simulink model "yoyo3"  (R2013b)
settings: Solver=ode45  StartTime=0.0  StopTime=10.0  RelTol=1e-3
values from neighbouring files (symbols this model uses):
  H = 1    [yoyo_model.m]    (also in yoyo_model_simulate.m = -100; yoyo_model_testing_lqi.m)
  K = 1    [yoyo_model.m]    (also in yoyo_model_simulate.m = 0.001; yoyo_model_testing_lqi.m)
  phi = fPHI(T,2*T,PARAMS)    [yoyo_model.m]    (also in yoyo_model_simulate.m; yoyo_model_testing_lqi.m = 1)
  psi = P.m * P.g * P.r / (P.epsilon * P.beta) * (exp(-P.beta * tf) - 2 * exp(-P.beta * (tf - tc)) - 1) - (P.m * P.g * P.r / P.epsilon) * tf    [fPSI.m]    (also in yoyo_model.m = fPSI(T,2*T,PARAMS); yoyo_model_simulate.m = fPSI(T,2*T,PARAMS); yoyo_model_testing_lqi.m = -100)
  yr = 0    [yoyo_model.m]    (also in yoyo_model_simulate.m; yoyo_model_testing_lqi.m)
settings Model: Creator=thomasesch  LastModifiedBy=thomasesch

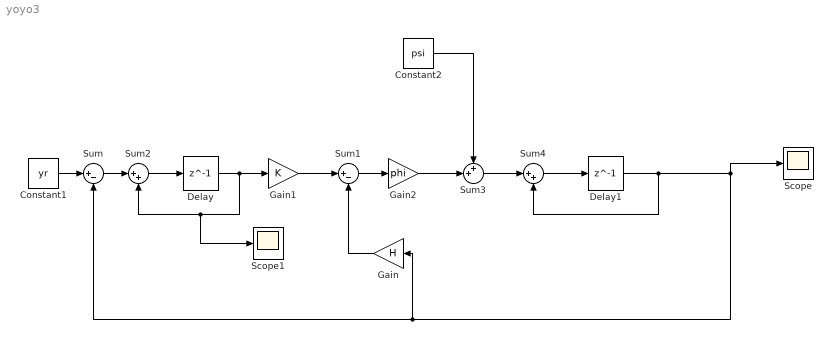
== system yoyo3 ==
  Constant1 : Constant  Value=yr
  Constant2 : Constant  Value=psi
  Delay : Delay  DelayLength=1  SampleTime=1
  Delay1 : Delay  DelayLength=1
  Gain : Gain  Gain=H
  Gain1 : Gain  Gain=K
  Gain2 : Gain  Gain=phi
  Scope : Scope
  Scope1 : Scope
  Sum : Sum  Inputs=|+-
  Sum1 : Sum  Inputs=|+-
  Sum2 : Sum  Inputs=|++
  Sum3 : Sum  Inputs=++|
  Sum4 : Sum  Inputs=|++
  wires:
  Sum4/1 -> Delay1/1
  Constant1/1 -> Sum/1
  Sum/1 -> Sum2/1
  Sum2/1 -> Delay/1
  Delay/1 -> Scope1/1, Sum2/2, Gain1/1
  Gain1/1 -> Sum1/1
  Gain/1 -> Sum1/2
  Constant2/1 -> Sum3/1
  Gain2/1 -> Sum3/2
  Sum1/1 -> Gain2/1
  Sum3/1 -> Sum4/1
  Delay1/1 -> Sum4/2, Gain/1, Sum/2, Scope/1
